simulink model "progStateFeedbackSim"  (R2018b)
settings: Solver=ode45  StartTime=0.0  StopTime=10.0  MaxStep=0.005  RelTol=1e-3  EnableMultiTasking=on
values from neighbouring files (symbols this model uses):
  A = [0 1 0; 0 -1 1; 0 0 -5]    [main.m]
  B = [0 0 5]'    [main.m]
  C = [1 0 0]    [main.m]
  Kacker = -acker(A,B,eig_cl_des)    [progStateFeedback (1).m]
  n = size(A,1)    [main.m]
  x0 = [2 1 0]    [main.m]
settings Model: Creator=roberto  LastModifiedBy=roberto
settings DataIOCC: LimitDataPoints=on  SaveFormat=Array
settings OptimizationCC: LifeSpan=inf
settings DebuggingCC: SFUnexpectedBacktrackingDiag=warning  SFNoUnconditionalDefaultTransitionDiag=warning  SFExecutionAtInitializationDiag=none
settings HardwareCC: ProdBitPerPointer=32  ProdBitPerSizeT=32  ProdBitPerPtrDiffT=32  ProdLargestAtomicFloat=None  ProdIntDivRoundTo=Undefined  ProdEndianess=Unspecified  ProdWordSize=32  ProdHWDeviceType=32-bit Generic
settings ModelReferenceCC: PropagateSignalLabelsOutOfModel=off
settings SFSimCC: SimUseLocalCustomCode=off
settings RTWCC: RTWUseLocalCustomCode=off
settings CodeAppCC: StateflowObjectComments=on
settings GRTTargetCC: TargetLangStandard=C89/C90 (ANSI)  GeneratePreprocessorConditionals=Disable all
settings ConfigComp: CovMetricSettings=dw  CovHtmlReporting=on  CovSaveCumulativeToWorkspaceVar=on  CovSaveSingleToWorkspaceVar=on  CovExternalEMLEnable=off

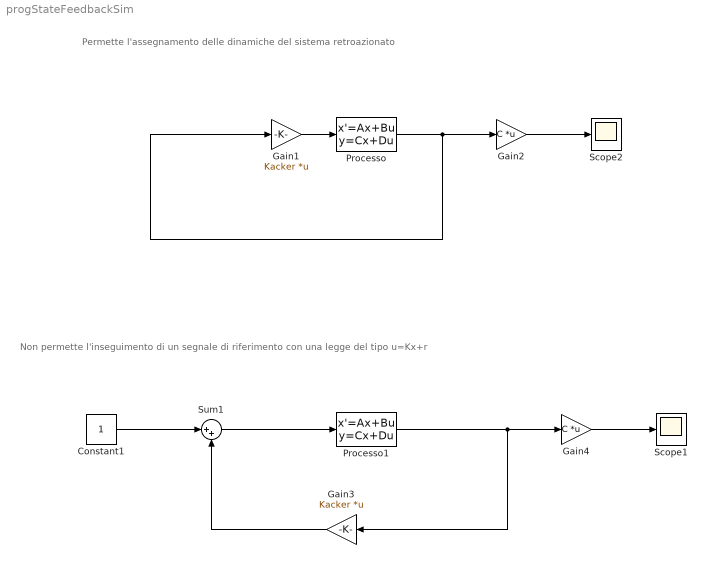
== system progStateFeedbackSim ==
  note: Permette l'assegnamento delle dinamiche del sistema retroazionato
  note: Non permette l'inseguimento di un segnale di riferimento con una legge del tipo u=Kx+r
  Constant1 : Constant
  Gain1 : Gain  Gain=Kacker  Multiplication=Matrix(K*u)
  Gain2 : Gain  Gain=C  Multiplication=Matrix(K*u)
  Gain3 : Gain  Gain=Kacker  Multiplication=Matrix(K*u)
  Gain4 : Gain  Gain=C  Multiplication=Matrix(K*u)
  Processo : StateSpace  A=A  B=B  C=eye(n)  D=zeros(n,1)  InitialCondition=x0
  Processo1 : StateSpace  A=A  B=B  C=eye(n)  D=zeros(n,1)  InitialCondition=x0*0
  Scope1 : Scope
  Scope2 : Scope
  Sum1 : Sum  Inputs=|++
  wires:
  Processo/1 -> Gain1/1, Gain2/1
  Gain1/1 -> Processo/1
  Gain2/1 -> Scope2/1
  Constant1/1 -> Sum1/1
  Processo1/1 -> Gain3/1, Gain4/1
  Sum1/1 -> Processo1/1
  Gain4/1 -> Scope1/1
  Gain3/1 -> Sum1/2
